simulink model "QPSK_sim"  (R2016b)
settings: Solver=ode45  StartTime=0  StopTime=30*Tsymb  MaxStep=1  RelTol=1e-3  EnableMultiTasking=on
values from neighbouring files (symbols this model uses):
  Beta = 0.2    [QPSK.m]
  BW_LPF = BW_CH    (= 0.0078125)    [QPSK.m]
  C_aprox = [1.60695392426680e-05 2.95841123026030e-05 5.48262790927617e-05 9.19832588239474e-05 0.000143686658983094 0.000212359882657570 0.000299965229015387 0.000407761225657029 0.000536071876123679 0.000684099631525166 0.000849796105711060 0.00102983168952252 0.00121960996869630 0.00141347333081234 0.00160490224533182 0.00178687182515771 0.00195224251942712 0.00209417001193910 0.00220655685058343 0.002284 ...(+463 chars)    [QPSK.m]
  C_aprox_err = C_aprox    [QPSK.m]
  fc = 1e6    (= 1000000)    [QPSK.m]    (also in ber.m; txrx.m)
  Samples_N = Tsymb/Te    [QPSK.m]
  Te = 1/fe    (= 1)    [QPSK.m]    (also in Trace_RC.m)
  Tsymb = round((1/BW_CH)*(1+Beta)*Te/2)    [QPSK.m]
libraries: commfilt2 x3, commrandsrc2 x2, simulink_extras x2, dspsigops x2, dspquant2 x2
settings Model: Creator=Solomesta  LastModifiedBy=charles
settings DataIOCC: LimitDataPoints=on  SaveFormat=Array
settings OptimizationCC: LifeSpan=inf
settings DebuggingCC: SolverPrmCheckMsg=warning  SFUnexpectedBacktrackingDiag=warning  SFNoUnconditionalDefaultTransitionDiag=warning  SFExecutionAtInitializationDiag=none
settings HardwareCC: ProdBitPerPointer=32  ProdBitPerSizeT=32  ProdBitPerPtrDiffT=32  ProdLargestAtomicFloat=None  ProdIntDivRoundTo=Undefined  ProdEndianess=Unspecified  ProdWordSize=32  ProdHWDeviceType=32-bit Generic
settings ModelReferenceCC: PropagateSignalLabelsOutOfModel=off
settings GRTTargetCC: TargetLangStandard=C89/C90 (ANSI)  GeneratePreprocessorConditionals=Disable all
settings ConfigComp: CovMetricSettings=dw  CovHtmlReporting=on  CovSaveCumulativeToWorkspaceVar=on  CovSaveSingleToWorkspaceVar=on  CovExternalEMLEnable=off  CovSFcnEnable=off

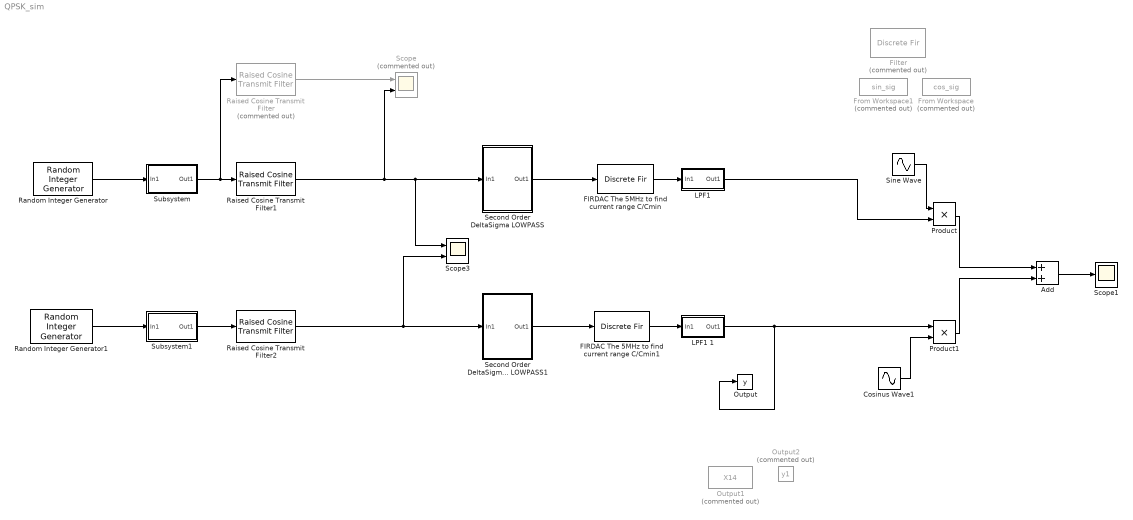
== system QPSK_sim ==
  " LPF1 " : Subsystem
  " LPF1 1" : Subsystem
  Add : Sum
  Cosinus Wave1 : Sin  Frequency=fc  SampleTime=0
  FIRDAC The 5MHz to find current range C/Cmin : DiscreteFir  Tag=BlockMethodSubSystem  Coefficients=C_aprox  InputProcessing=Columns as channels (frame based)  SampleTime=Te
  FIRDAC The 5MHz to find current range C/Cmin1 : DiscreteFir  Tag=BlockMethodSubSystem  Coefficients=C_aprox_err  InputProcessing=Columns as channels (frame based)  SampleTime=Te
  Filter : DiscreteFir  Tag=BlockMethodSubSystem  Commented=on  Coefficients=[0.00031396486105330918 0.00079428285105145966 0.0016984460144757131 0.003147515761969001 0.005273983695907117 0.0081755969271476957 0.011890632023848853 0.016376635112121077 0.021497899106786685 0.027023963192893654 0.032642275312797751 0.037984217148575632 0.042661300834204628 0.046308915935646247 0.048628459074510078 0.049424377526171376 0.048628459074510078 0.046308915935646247 0.042661300834204628 0.037984217148575632 0.032642275312797751 0.027023963192893654 0.021497899106786685 0.016376635112121077 0.011890632023848853 0.0081755969271476957 0.005273983695907117 0.003147515761969001 0.0016984460144757131 0.00079428285105145966 0.00031396486105330918]  InputProcessing=Columns as channels (frame based)
  From Workspace : FromWorkspace  Commented=on  VariableName=cos_sig  SampleTime=1
  From Workspace1 : FromWorkspace  Commented=on  VariableName=sin_sig  SampleTime=1
  Output : ToWorkspace  VariableName=y  SampleTime=1
      settings: MaxDataPoints=N
  Output1 : ToWorkspace  Commented=on  VariableName=X14  SampleTime=1
      settings: MaxDataPoints=N
  Output2 : ToWorkspace  Commented=on  VariableName=y1  SampleTime=1
      settings: MaxDataPoints=N
  Product : Product
  Product1 : Product
  Raised Cosine Transmit Filter : commfilt2/Raised Cosine Transmit Filter  Commented=on  filtType=Normal  R=Beta  filtSpan=2  N=Samples_N  filterGain=1  InputProcessing=Columns as channels (frame based)  RateOptions=Allow multirate processing  framing=Mute  checkCoeff=off  variableName=rcTxFilt  checkGain=Normalized  sampMode=Mute  saveAsFlag=0  currentFiltSpan=2  D=(2)/2  launchFVT=on  roundingMode=Floor  overflowMode=off  coeffDataTypeStr=Inherit: Same word length as input  coeffMin=[]  coeffMax=[]  coeffLastDataTypeStr=Inherit: Same word length as input  outputDataTypeStr=Inherit: Same as accumulator  outputMin=[]  outputMax=[]  outputLastDataTypeStr=Inherit: Same as accumulator
  Raised Cosine Transmit Filter1 : commfilt2/Raised Cosine Transmit Filter  filtType=Normal  R=Beta  filtSpan=2  N=Samples_N  filterGain=1  InputProcessing=Columns as channels (frame based)  RateOptions=Allow multirate processing  framing=Mute  checkCoeff=off  variableName=rcTxFilt1  checkGain=Normalized  sampMode=Mute  saveAsFlag=0  currentFiltSpan=2  D=(2)/2  launchFVT=on  roundingMode=Floor  overflowMode=off  coeffDataTypeStr=Inherit: Same word length as input  coeffMin=[]  coeffMax=[]  coeffLastDataTypeStr=Inherit: Same word length as input  outputDataTypeStr=Inherit: Same as accumulator  outputMin=[]  outputMax=[]  outputLastDataTypeStr=Inherit: Same as accumulator
  Raised Cosine Transmit Filter2 : commfilt2/Raised Cosine Transmit Filter  filtType=Normal  R=Beta  filtSpan=2  N=Samples_N  filterGain=1  InputProcessing=Columns as channels (frame based)  RateOptions=Allow multirate processing  framing=Mute  checkCoeff=off  variableName=rcTxFilt2  checkGain=Normalized  sampMode=Mute  saveAsFlag=0  currentFiltSpan=2  D=(2)/2  launchFVT=on  roundingMode=Floor  overflowMode=off  coeffDataTypeStr=Inherit: Same word length as input  coeffMin=[]  coeffMax=[]  coeffLastDataTypeStr=Inherit: Same word length as input  outputDataTypeStr=Inherit: Same as accumulator  outputMin=[]  outputMax=[]  outputLastDataTypeStr=Inherit: Same as accumulator
  Random Integer Generator : commrandsrc2/Random Integer Generator  mul=2  seed=37  Ts=Tsymb  frameBased=off  sampPerFrame=1  orient=off  outDataType=double
  Random Integer Generator1 : commrandsrc2/Random Integer Generator  mul=2  seed=3000  Ts=Tsymb  frameBased=off  sampPerFrame=1  orient=off  outDataType=double
  Scope : Scope  Commented=on  NumInputPorts=2
  Scope1 : Scope
  Scope3 : Scope  NumInputPorts=2
  Second Order DeltaSigma LOWPASS : Subsystem
  Second Order DeltaSigma LOWPASS1 : Subsystem
  Sine Wave : Sin  Amplitude=sqrt(2/Tsymb)  Frequency=fc  Phase=pi/2  SampleTime=0
  Subsystem : Subsystem
  Subsystem1 : Subsystem
  wires:
  Random Integer Generator/1 -> Subsystem/1(In1)
  Subsystem/1(Out1) -> Raised Cosine Transmit Filter1/1, Raised Cosine Transmit Filter/1
  Raised Cosine Transmit Filter/1 -> Scope/1
  Second Order DeltaSigma LOWPASS/1(Out1) -> FIRDAC The 5MHz to find current range C/Cmin/1
  FIRDAC The 5MHz to find current range C/Cmin/1 -> " LPF1 "/1(In1)
  Second Order DeltaSigma LOWPASS1/1(Out1) -> FIRDAC The 5MHz to find current range C/Cmin1/1
  FIRDAC The 5MHz to find current range C/Cmin1/1 -> " LPF1 1"/1(In1)
  Raised Cosine Transmit Filter2/1 -> Scope3/2, Second Order DeltaSigma LOWPASS1/1(In1)
  Subsystem1/1(Out1) -> Raised Cosine Transmit Filter2/1
  Random Integer Generator1/1 -> Subsystem1/1(In1)
  Raised Cosine Transmit Filter1/1 -> Scope/2, Scope3/1, Second Order DeltaSigma LOWPASS/1(In1)
  Product1/1 -> Add/2
  Product/1 -> Add/1
  Sine Wave/1 -> Product/1
  Cosinus Wave1/1 -> Product1/2
  Add/1 -> Scope1/1
  " LPF1 "/1(Out1) -> Product/2
  " LPF1 1"/1(Out1) -> Product1/1, Output/1

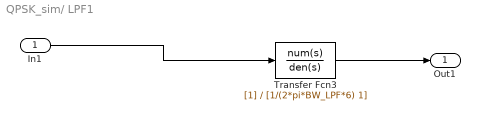
== system QPSK_sim/ LPF1  ==
  In1 : Inport
  Transfer Fcn3 : TransferFcn  Denominator=[1/(2*pi*BW_LPF*6) 1]
  Out1 : Outport
  wires:
  In1/1 -> Transfer Fcn3/1
  Transfer Fcn3/1 -> Out1/1

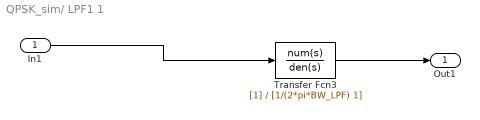
== system QPSK_sim/ LPF1 1 ==
  In1 : Inport
  Transfer Fcn3 : TransferFcn  Denominator=[1/(2*pi*BW_LPF) 1]
  Out1 : Outport
  wires:
  In1/1 -> Transfer Fcn3/1
  Transfer Fcn3/1 -> Out1/1

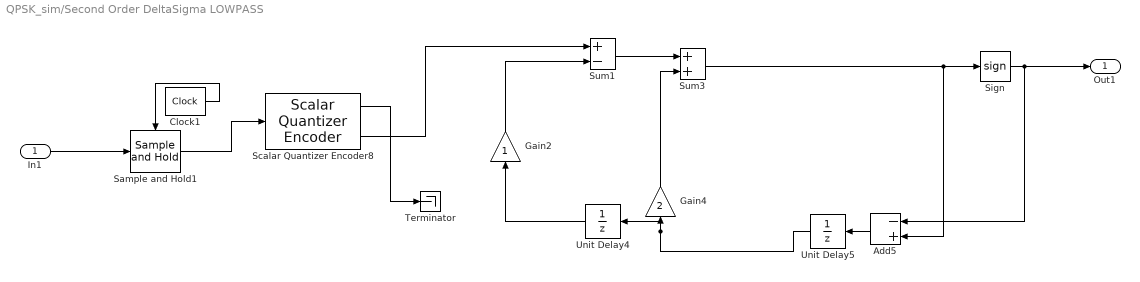
== system QPSK_sim/Second Order DeltaSigma LOWPASS ==
  In1 : Inport
  Add5 : Sum  Inputs=-+  SampleTime=Te
  Clock1 : simulink_extras/Flip Flops/Clock  period=Te
  Gain2 : Gain  SampleTime=Te
  Gain4 : Gain  Gain=2  SampleTime=Te
  Sample and Hold1 : dspsigops/Sample and Hold  trig=Rising edge  initCond=0  latchinput=off
  Scalar Quantizer Encoder8 : dspquant2/Scalar Quantizer Encoder  paramSrc=Specify via dialog  partType=Bounded  BBoundary=Bound1  UBoundary=[2:9]  SearchMethod=Linear  tieBreakRule=Choose the lower index  outQU=on  outQError=off  codebook=code1  outStatus=off  invalidin=Clip  idtype=int32  roundingMode=Floor  overflowMode=off
  Sign : Signum  SampleTime=Te
  Sum1 : Sum  Inputs=+-  SampleTime=Te  SaturateOnIntegerOverflow=on  InputSameDT=on  OutDataTypeStr=Inherit: Same as first input
  Sum3 : Sum  SampleTime=Te  SaturateOnIntegerOverflow=on  InputSameDT=on  OutDataTypeStr=Inherit: Same as first input
  Terminator : Terminator
  Unit Delay4 : UnitDelay  SampleTime=Te
  Unit Delay5 : UnitDelay  SampleTime=Te
  Out1 : Outport
  wires:
  Scalar Quantizer Encoder8/2 -> Sum1/1
  Unit Delay4/1 -> Gain2/1
  In1/1 -> Sample and Hold1/1
  Clock1/1 -> Sample and Hold1/Trigger
  Sum3/1 -> Add5/2, Sign/1
  Add5/1 -> Unit Delay5/1
  Sign/1 -> Out1/1, Add5/1
  Sample and Hold1/1 -> Scalar Quantizer Encoder8/1
  Unit Delay5/1 -> Unit Delay4/1, Gain4/1
  Gain2/1 -> Sum1/2
  Gain4/1 -> Sum3/2
  Sum1/1 -> Sum3/1
  Scalar Quantizer Encoder8/1 -> Terminator/1

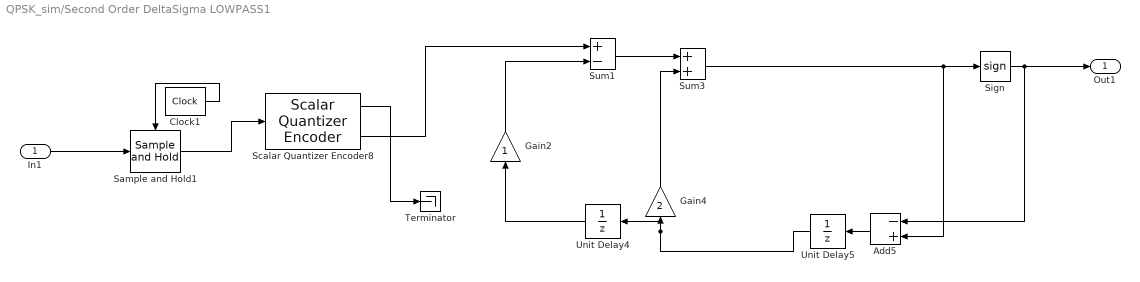
== system QPSK_sim/Second Order DeltaSigma LOWPASS1 ==
  In1 : Inport
  Add5 : Sum  Inputs=-+  SampleTime=Te
  Clock1 : simulink_extras/Flip Flops/Clock  period=Te
  Gain2 : Gain  SampleTime=Te
  Gain4 : Gain  Gain=2  SampleTime=Te
  Sample and Hold1 : dspsigops/Sample and Hold  trig=Rising edge  initCond=0  latchinput=off
  Scalar Quantizer Encoder8 : dspquant2/Scalar Quantizer Encoder  paramSrc=Specify via dialog  partType=Bounded  BBoundary=Bound1  UBoundary=[2:9]  SearchMethod=Linear  tieBreakRule=Choose the lower index  outQU=on  outQError=off  codebook=code1  outStatus=off  invalidin=Clip  idtype=int32  roundingMode=Floor  overflowMode=off
  Sign : Signum  SampleTime=Te
  Sum1 : Sum  Inputs=+-  SampleTime=Te  SaturateOnIntegerOverflow=on  InputSameDT=on  OutDataTypeStr=Inherit: Same as first input
  Sum3 : Sum  SampleTime=Te  SaturateOnIntegerOverflow=on  InputSameDT=on  OutDataTypeStr=Inherit: Same as first input
  Terminator : Terminator
  Unit Delay4 : UnitDelay  SampleTime=Te
  Unit Delay5 : UnitDelay  SampleTime=Te
  Out1 : Outport
  wires:
  Scalar Quantizer Encoder8/2 -> Sum1/1
  Unit Delay4/1 -> Gain2/1
  In1/1 -> Sample and Hold1/1
  Clock1/1 -> Sample and Hold1/Trigger
  Sum3/1 -> Add5/2, Sign/1
  Add5/1 -> Unit Delay5/1
  Sign/1 -> Out1/1, Add5/1
  Sample and Hold1/1 -> Scalar Quantizer Encoder8/1
  Unit Delay5/1 -> Unit Delay4/1, Gain4/1
  Gain2/1 -> Sum1/2
  Gain4/1 -> Sum3/2
  Sum1/1 -> Sum3/1
  Scalar Quantizer Encoder8/1 -> Terminator/1

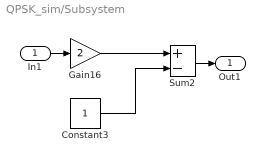
== system QPSK_sim/Subsystem ==
  In1 : Inport
  Constant3 : Constant  SampleTime=-1
  Gain16 : Gain  Gain=2
  Sum2 : Sum  Inputs=+-  SaturateOnIntegerOverflow=on  InputSameDT=on  OutDataTypeStr=Inherit: Same as first input
  Out1 : Outport
  wires:
  Constant3/1 -> Sum2/2
  Gain16/1 -> Sum2/1
  Sum2/1 -> Out1/1
  In1/1 -> Gain16/1

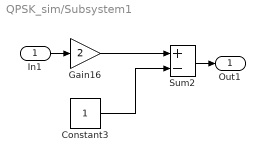
== system QPSK_sim/Subsystem1 ==
  In1 : Inport
  Constant3 : Constant  SampleTime=-1
  Gain16 : Gain  Gain=2
  Sum2 : Sum  Inputs=+-  SaturateOnIntegerOverflow=on  InputSameDT=on  OutDataTypeStr=Inherit: Same as first input
  Out1 : Outport
  wires:
  Constant3/1 -> Sum2/2
  Gain16/1 -> Sum2/1
  Sum2/1 -> Out1/1
  In1/1 -> Gain16/1
